simulink model "youbot_EC_flat_45_with_flexibility"  (R2017b)
settings: Solver=VariableStepAuto  StartTime=0.0  StopTime=3  MaxStep=0.01  RelTol=1e-4  EnableMultiTasking=on
values from neighbouring files (symbols this model uses):
  B_env = 1.8    [motor_model_kuka_youbot.m]    (also in motor_model_kuka_youbot2.m = 0.01)
  B_m = 23e-3    (= 0.023)    [motor_model_kuka_youbot2.m]
  J = Jm + 1/(N^2)*(Jr + Jch)    (= 1.2077288055e-05)    [motor_model_kuka_youbot.m]    (also in motor_model_kuka_youbot2.m = 0.000181)
  J_rob = 661e-6    (= 0.000661)    [motor_model_kuka_youbot2.m]
  K = k    (= 10)    [motor_model_kuka_youbot.m]    (also in motor_model_kuka_youbot2.m = i/1000)
  K_cur = Ki    (= 3.54813389234)    [Untitled.m]    (also in motor_model_kuka_youbot.m = 3000; motor_model_kuka_youbot2.m = 11.71875)
  K_env = 25    [motor_model_kuka_youbot.m]    (also in motor_model_kuka_youbot2.m = 1)
  K_m = 31e-1    (= 3.1)    [motor_model_kuka_youbot2.m]
  Ke = 51.1e-3    (= 0.0511)    [motor_model_kuka_youbot.m]    (also in motor_model_kuka_youbot2.m = 1.10867309417)
  kf = R*Jm/L * 1e-6    (= 1.85e-11)    [motor_model_kuka_youbot.m]    (also in motor_model_kuka_youbot2.m = 0.000237684665227)
  Ki = 10^(11/20)    (= 3.54813389234)    [Untitled.m]    (also in motor_model_kuka_youbot.m = 1; motor_model_kuka_youbot2.m = j/1000)
  Ki_cur = Ki/Ti    (= 17740.6694617)    [Untitled.m]    (also in motor_model_kuka_youbot.m = 3000; motor_model_kuka_youbot2.m = 0.0114440917969)
  Kt = 51e-3    (= 0.051)    [motor_model_kuka_youbot.m]    (also in motor_model_kuka_youbot2.m = 0.0369)
  Kv = 200    [motor_model_kuka_youbot.m]    (also in motor_model_kuka_youbot2.m = 0.78125)
  L = 2.24    [motor_model_kuka_youbot.m]    (also in motor_model_kuka_youbot2.m = 0.000463)
  R = 4.48    [motor_model_kuka_youbot.m]    (also in motor_model_kuka_youbot2.m = 0.608)
  tau_e = L/(3*R)    (= 0.166666666667)    [motor_model_kuka_youbot.m]    (also in motor_model_kuka_youbot2.m = 0.000253837719298)
  tau_m = 11.8e-3    (= 0.0118)    [motor_model_kuka_youbot.m]    (also in motor_model_kuka_youbot2.m = 0.00807)
libraries: simulink x3
settings Model: Creator=fortineau_vin  LastModifiedBy=fortineau_vin
settings DataIOCC: LimitDataPoints=on  SaveOutput=off  SaveTime=off
settings OptimizationCC: ExpressionDepthLimit=2147483647  LifeSpan=1
settings DebuggingCC: UnderspecifiedInitializationDetection=Classic  MergeDetectMultiDrivingBlocksExec=none  FcnCallInpInsideContextMsg=warning  AllowSymbolicDim=off  StateNameClashWarn=warning  SFUnexpectedBacktrackingDiag=warning  SFNoUnconditionalDefaultTransitionDiag=warning  SFExecutionAtInitializationDiag=none
settings CodeAppCC: StateflowObjectComments=on
settings GRTTargetCC: TargetLangStandard=C89/C90 (ANSI)  GeneratePreprocessorConditionals=Disable all  CombineOutputUpdateFcns=off  GRTInterface=on

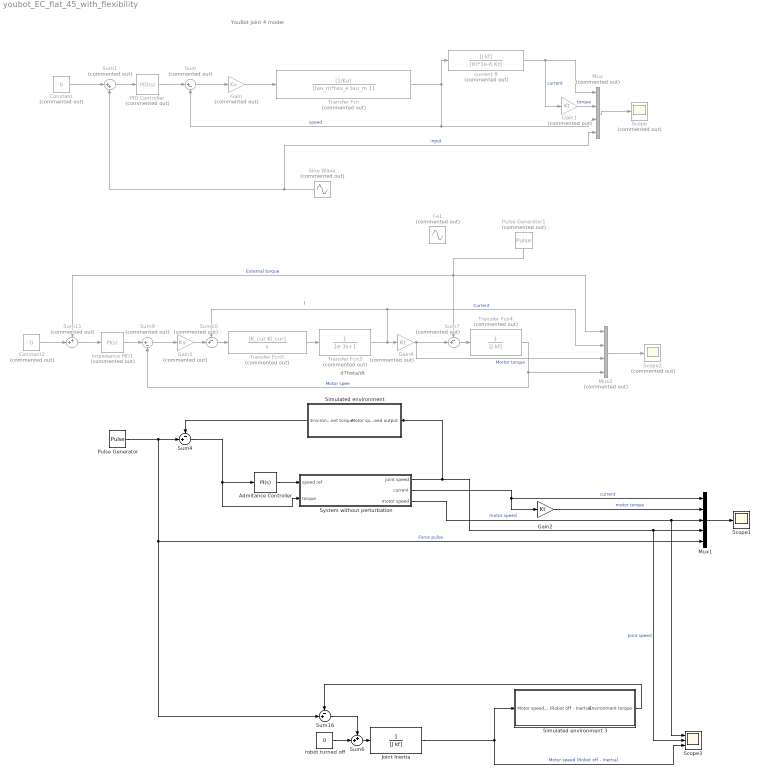
== system youbot_EC_flat_45_with_flexibility ==
  note: YouBot joint 4 model
  note: I
  note: dTheta/dt
  Admitance Controller : simulink/Continuous/PID Controller  Controller=PI  TimeDomain=Continuous-time  SampleTime=-1  IntegratorMethod=Forward Euler  FilterMethod=Forward Euler  Form=Parallel  UseFilter=on  ControllerParametersSource=internal  P=K  I=Ki  D=0  N=0  InitialConditionSource=internal  InitialConditionForIntegrator=0  InitialConditionForFilter=0  ExternalReset=none  LimitOutput=off  UpperSaturationLimit=inf  LowerSaturationLimit=-inf  LinearizeAsGain=on  AntiWindupMode=none  Kb=1  TrackingMode=off  Kt=1  PParamMin=[]  PParamMax=[]  IParamMin=[]  IParamMax=[]  DParamMin=[]  DParamMax=[]  NParamMin=[]  NParamMax=[]  KbParamMin=[]  KbParamMax=[]  KtParamMin=[]  KtParamMax=[]  POutMin=[]  POutMax=[]  IOutMin=[]  IOutMax=[]  DOutMin=[]  DOutMax=[]  NOutMin=[]  NOutMax=[]  KbOutMin=[]  KbOutMax=[]  KtOutMin=[]  KtOutMax=[]  IntegratorOutMin=[]  IntegratorOutMax=[]  FilterOutMin=[]  FilterOutMax=[]  SumOutMin=[]  SumOutMax=[]  SumI1OutMin=[]  SumI1OutMax=[]  SumI2OutMin=[]  SumI2OutMax=[]  SumI3OutMin=[]  SumI3OutMax=[]  SumDOutMin=[]  SumDOutMax=[]  SaturationOutMin=[]  SaturationOutMax=[]  IntegratorContinuousStateAttributes=''  IntegratorStateMustResolveToSignalObject=off  IntegratorRTWStateStorageClass=Auto  FilterContinuousStateAttributes=''  FilterStateMustResolveToSignalObject=off  FilterRTWStateStorageClass=Auto  DifferentiatorICPrevScaledInput=0  DifferentiatorOutMin=[]  DifferentiatorOutMax=[]  InitialConditionSetting=State (most efficient)  FilterDiffOutCoefMin=[]  FilterDiffOutCoefMax=[]  SumDenOutMin=[]  SumDenOutMax=[]  SumNumOutMin=[]  SumNumOutMax=[]  ReciprocalOutMin=[]  ReciprocalOutMax=[]  DivideOutMin=[]  DivideOutMax=[]  TunerSelectOption=Transfer Function Based (PID Tuner App)
  Constant : Constant  Commented=on  Value=0
  Constant2 : Constant  Commented=on  Value=0
  Fe1 : Sin  Commented=on  Amplitude=5  Frequency=0.1*(2*pi)  Samples=100  SampleTime=0
  Gain : Gain  Commented=on  Gain=Kv
  Gain1 : Gain  Commented=on  Gain=Kt
  Gain2 : Gain  Gain=Kt
  Gain4 : Gain  Commented=on  Gain=Kt
  Gain5 : Gain  Commented=on  Gain=Kv
  Joint Inertia : TransferFcn  Denominator=[J kf]
  Mux : Mux  Commented=on
  Mux1 : Mux  Inputs=5
  Mux2 : Mux  Commented=on
  PID Controller : simulink/Continuous/PID Controller  Commented=on  Controller=PID  TimeDomain=Continuous-time  SampleTime=-1  IntegratorMethod=Forward Euler  FilterMethod=Forward Euler  Form=Parallel  UseFilter=on  ControllerParametersSource=internal  P=K  I=Ki  D=0  N=0  InitialConditionSource=internal  InitialConditionForIntegrator=0  InitialConditionForFilter=0  ExternalReset=none  LimitOutput=off  UpperSaturationLimit=inf  LowerSaturationLimit=-inf  LinearizeAsGain=on  AntiWindupMode=none  Kb=1  TrackingMode=off  Kt=1  PParamMin=[]  PParamMax=[]  IParamMin=[]  IParamMax=[]  DParamMin=[]  DParamMax=[]  NParamMin=[]  NParamMax=[]  KbParamMin=[]  KbParamMax=[]  KtParamMin=[]  KtParamMax=[]  POutMin=[]  POutMax=[]  IOutMin=[]  IOutMax=[]  DOutMin=[]  DOutMax=[]  NOutMin=[]  NOutMax=[]  KbOutMin=[]  KbOutMax=[]  KtOutMin=[]  KtOutMax=[]  IntegratorOutMin=[]  IntegratorOutMax=[]  FilterOutMin=[]  FilterOutMax=[]  SumOutMin=[]  SumOutMax=[]  SumI1OutMin=[]  SumI1OutMax=[]  SumI2OutMin=[]  SumI2OutMax=[]  SumI3OutMin=[]  SumI3OutMax=[]  SumDOutMin=[]  SumDOutMax=[]  SaturationOutMin=[]  SaturationOutMax=[]  IntegratorContinuousStateAttributes=''  IntegratorStateMustResolveToSignalObject=off  IntegratorRTWStateStorageClass=Auto  FilterContinuousStateAttributes=''  FilterStateMustResolveToSignalObject=off  FilterRTWStateStorageClass=Auto  DifferentiatorICPrevScaledInput=0  DifferentiatorOutMin=[]  DifferentiatorOutMax=[]  InitialConditionSetting=State (most efficient)  FilterDiffOutCoefMin=[]  FilterDiffOutCoefMax=[]  SumDenOutMin=[]  SumDenOutMax=[]  SumNumOutMin=[]  SumNumOutMax=[]  ReciprocalOutMin=[]  ReciprocalOutMax=[]  DivideOutMin=[]  DivideOutMax=[]  TunerSelectOption=Transfer Function Based (PID Tuner App)
  Pulse Generator : DiscretePulseGenerator  PulseType=Time based  Period=0.5  PulseWidth=25
  Pulse Generator1 : DiscretePulseGenerator  Commented=on  PulseType=Time based  Period=0.5  PulseWidth=25
  Scope : Scope  Commented=on
  Scope1 : Scope
  Scope2 : Scope  Commented=on
  Scope3 : Scope  NumInputPorts=3
  Simulated environment : Subsystem
  Simulated environment 3 : Subsystem
  Sine Wave : Sin  Commented=on  Amplitude=5  Frequency=10  SampleTime=0
  Sum : Sum  Commented=on  Inputs=|+-
  Sum1 : Sum  Commented=on  Inputs=|++
  Sum10 : Sum  Commented=on  Inputs=-+|
  Sum11 : Sum  Commented=on  Inputs=++|
  Sum16 : Sum  Inputs=-+|
  Sum4 : Sum  Inputs=-+|
  Sum6 : Sum  Inputs=++|
  Sum7 : Sum  Commented=on  Inputs=-+|
  Sum9 : Sum  Commented=on  Inputs=|+-
  System without perturbation : Subsystem
  Transfer Fcn : TransferFcn  Commented=on  Numerator=[1/Ke]  Denominator=[tau_m*tau_e tau_m 1]
  Transfer Fcn3 : TransferFcn  Commented=on  Denominator=[1e-3 1]
  Transfer Fcn4 : TransferFcn  Commented=on  Denominator=[J kf]
  Transfer Fcn5 : TransferFcn  Commented=on  Numerator=[K_cur Ki_cur]  Denominator=[1 0]
  current ft : TransferFcn  Commented=on  Numerator=[J kf]  Denominator=[Kt*1e-6 Kt]
  impedance PID1 : simulink/Continuous/PID Controller  Commented=on  Controller=PI  TimeDomain=Continuous-time  SampleTime=-1  IntegratorMethod=Forward Euler  FilterMethod=Forward Euler  Form=Parallel  UseFilter=on  ControllerParametersSource=internal  P=K  I=Ki  D=0  N=0  InitialConditionSource=internal  InitialConditionForIntegrator=0  InitialConditionForFilter=0  ExternalReset=none  LimitOutput=off  UpperSaturationLimit=inf  LowerSaturationLimit=-inf  LinearizeAsGain=on  AntiWindupMode=none  Kb=1  TrackingMode=off  Kt=1  PParamMin=[]  PParamMax=[]  IParamMin=[]  IParamMax=[]  DParamMin=[]  DParamMax=[]  NParamMin=[]  NParamMax=[]  KbParamMin=[]  KbParamMax=[]  KtParamMin=[]  KtParamMax=[]  POutMin=[]  POutMax=[]  IOutMin=[]  IOutMax=[]  DOutMin=[]  DOutMax=[]  NOutMin=[]  NOutMax=[]  KbOutMin=[]  KbOutMax=[]  KtOutMin=[]  KtOutMax=[]  IntegratorOutMin=[]  IntegratorOutMax=[]  FilterOutMin=[]  FilterOutMax=[]  SumOutMin=[]  SumOutMax=[]  SumI1OutMin=[]  SumI1OutMax=[]  SumI2OutMin=[]  SumI2OutMax=[]  SumI3OutMin=[]  SumI3OutMax=[]  SumDOutMin=[]  SumDOutMax=[]  SaturationOutMin=[]  SaturationOutMax=[]  IntegratorContinuousStateAttributes=''  IntegratorStateMustResolveToSignalObject=off  IntegratorRTWStateStorageClass=Auto  FilterContinuousStateAttributes=''  FilterStateMustResolveToSignalObject=off  FilterRTWStateStorageClass=Auto  DifferentiatorICPrevScaledInput=0  DifferentiatorOutMin=[]  DifferentiatorOutMax=[]  InitialConditionSetting=State (most efficient)  FilterDiffOutCoefMin=[]  FilterDiffOutCoefMax=[]  SumDenOutMin=[]  SumDenOutMax=[]  SumNumOutMin=[]  SumNumOutMax=[]  ReciprocalOutMin=[]  ReciprocalOutMax=[]  DivideOutMin=[]  DivideOutMax=[]  TunerSelectOption=Transfer Function Based (PID Tuner App)
  robot turned off : Constant  Value=0
  wires:
  Transfer Fcn/1 -> current ft/1, Mux/3, Sum/2  "speed"
  Gain/1 -> Transfer Fcn/1
  Sum/1 -> Gain/1
  PID Controller/1 -> Sum/1
  Sum1/1 -> PID Controller/1
  Constant/1 -> Sum1/1
  Sine Wave/1 -> Mux/4, Sum1/2  "input"
  current ft/1 -> Gain1/1, Mux/1  "current"
  Gain1/1 -> Mux/2  "torque"
  Mux/1 -> Scope/1
  Mux2/1 -> Scope2/1
  Pulse Generator1/1 -> Sum11/1, Mux2/1, Sum7/1  "External torque"
  Constant2/1 -> Sum11/2
  Gain4/1 -> Sum7/2, Mux2/3  "Mortor torque"
  Transfer Fcn4/1 -> Mux2/4, Sum9/2  "Motor spee"
  Sum7/1 -> Transfer Fcn4/1
  impedance PID1/1 -> Sum9/1
  Transfer Fcn3/1 -> Gain4/1, Sum10/1, Mux2/2  "Current"
  Sum11/1 -> impedance PID1/1
  Gain5/1 -> Sum10/2
  Sum9/1 -> Gain5/1
  Sum10/1 -> Transfer Fcn5/1
  Transfer Fcn5/1 -> Transfer Fcn3/1
  System without perturbation/1(joint speed) -> Simulated environment/1(Motor speed output), Scope3/2, Mux1/4  "Joint speed"
  Admitance Controller/1 -> System without perturbation/1(speed ref)
  Pulse Generator/1 -> Sum4/2, Mux1/5, Sum16/2  "Force pulse"
  System without perturbation/2(current) -> Mux1/1, Gain2/1  "current"
  Gain2/1 -> Mux1/2  "motor torque"
  Sum4/1 -> System without perturbation/2(torque), Admitance Controller/1
  Sum6/1 -> Joint Inertia/1
  Joint Inertia/1 -> Simulated environment 3/1(Motor speed (Robot off - Inertia)), Scope3/3  "Motor speed (Robot off - Inertia)"
  Sum16/1 -> Sum6/1
  robot turned off/1 -> Sum6/2
  Simulated environment/1(Environment torque) -> Sum4/1
  Simulated environment 3/1(Environment torque) -> Sum16/1
  System without perturbation/3(motor speed) -> Scope3/1, Mux1/3  "motor speed"
  Mux1/1 -> Scope1/1

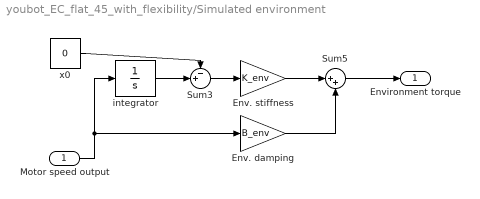
== system youbot_EC_flat_45_with_flexibility/Simulated environment ==
  Motor speed output : Inport
  Env. damping : Gain  Gain=B_env
  Env. stiffness : Gain  Gain=K_env
  Sum3 : Sum  Inputs=-+|
  Sum5 : Sum  Inputs=|++
  integrator : TransferFcn  Denominator=[1 0]
  x0 : Constant  Value=0
  Environment torque : Outport
  wires:
  integrator/1 -> Sum3/2
  x0/1 -> Sum3/1
  Sum3/1 -> Env. stiffness/1
  Sum5/1 -> Environment torque/1
  Env. damping/1 -> Sum5/2
  Env. stiffness/1 -> Sum5/1
  Motor speed output/1 -> Env. damping/1, integrator/1

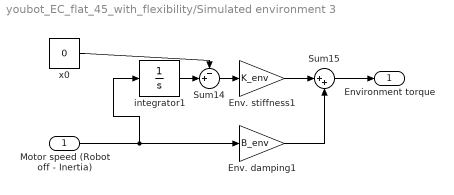
== system youbot_EC_flat_45_with_flexibility/Simulated environment 3 ==
  Motor speed (Robot off - Inertia) : Inport
  Env. damping1 : Gain  Gain=B_env
  Env. stiffness1 : Gain  Gain=K_env
  Sum14 : Sum  Inputs=-+|
  Sum15 : Sum  Inputs=|++
  integrator1 : TransferFcn  Denominator=[1 0]
  x0 : Constant  Value=0
  Environment torque : Outport
  wires:
  Env. stiffness1/1 -> Sum15/1
  integrator1/1 -> Sum14/2
  Sum14/1 -> Env. stiffness1/1
  x0/1 -> Sum14/1
  Env. damping1/1 -> Sum15/2
  Sum15/1 -> Environment torque/1
  Motor speed (Robot off - Inertia)/1 -> integrator1/1, Env. damping1/1

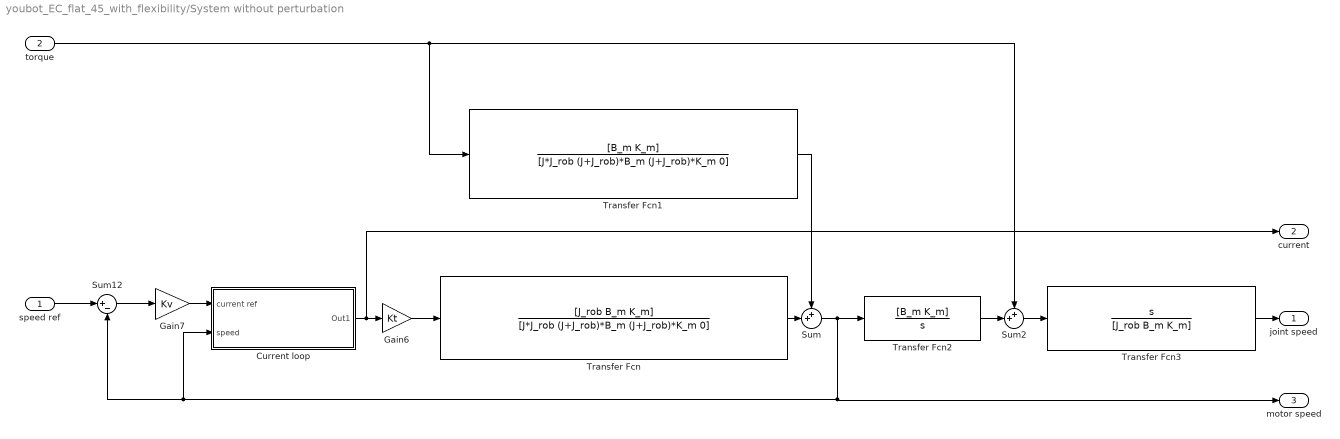
== system youbot_EC_flat_45_with_flexibility/System without perturbation ==
  speed ref : Inport
  torque : Inport  Port=2
  Current loop : Subsystem
  Gain6 : Gain  Gain=Kt
  Gain7 : Gain  Gain=Kv
  Sum : Sum  Inputs=++|
  Sum12 : Sum  Inputs=|+-
  Sum2 : Sum  Inputs=++|
  Transfer Fcn : TransferFcn  Numerator=[J_rob B_m K_m]  Denominator=[J*J_rob (J+J_rob)*B_m (J+J_rob)*K_m 0]
  Transfer Fcn1 : TransferFcn  Numerator=[B_m K_m]  Denominator=[J*J_rob (J+J_rob)*B_m (J+J_rob)*K_m 0]
  Transfer Fcn2 : TransferFcn  Numerator=[B_m K_m]  Denominator=[1 0]
  Transfer Fcn3 : TransferFcn  Numerator=[1 0]  Denominator=[J_rob B_m K_m]
  joint speed : Outport
  current : Outport  Port=2
  motor speed : Outport  Port=3
  wires:
  speed ref/1 -> Sum12/1
  Sum12/1 -> Gain7/1
  Sum/1 -> Transfer Fcn2/1, Sum12/2, Current loop/2(speed), motor speed/1
  Gain7/1 -> Current loop/1(current ref)
  Current loop/1(Out1) -> Gain6/1, current/1
  Gain6/1 -> Transfer Fcn/1
  Transfer Fcn/1 -> Sum/2
  Transfer Fcn1/1 -> Sum/1
  torque/1 -> Sum2/1, Transfer Fcn1/1
  Transfer Fcn2/1 -> Sum2/2
  Sum2/1 -> Transfer Fcn3/1
  Transfer Fcn3/1 -> joint speed/1

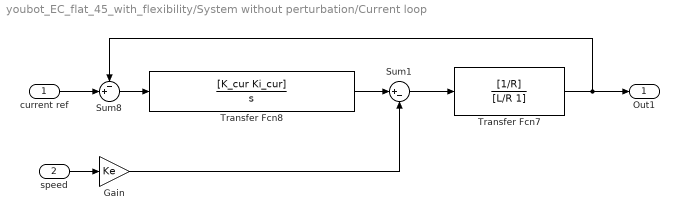
== system youbot_EC_flat_45_with_flexibility/System without perturbation/Current loop ==
  current ref : Inport
  speed : Inport  Port=2
  Gain : Gain  Gain=Ke
  Sum1 : Sum  Inputs=|+-
  Sum8 : Sum  Inputs=-+|
  Transfer Fcn7 : TransferFcn  Numerator=[1/R]  Denominator=[L/R 1]
  Transfer Fcn8 : TransferFcn  Numerator=[K_cur Ki_cur]  Denominator=[1 0]
  Out1 : Outport
  wires:
  Sum8/1 -> Transfer Fcn8/1
  Transfer Fcn7/1 -> Out1/1, Sum8/1
  current ref/1 -> Sum8/2
  Transfer Fcn8/1 -> Sum1/1
  speed/1 -> Gain/1
  Gain/1 -> Sum1/2
  Sum1/1 -> Transfer Fcn7/1
